simulink model "CTRL_UP_YAWACC_test"  (R2023b)
settings: Solver=VariableStepAuto  StartTime=0.0  StopTime=10.0  RelTol=1e-3
libraries: CTRL_UP_YAWACC x1
settings Model: Creator=blatak  LastModifiedBy=blatak

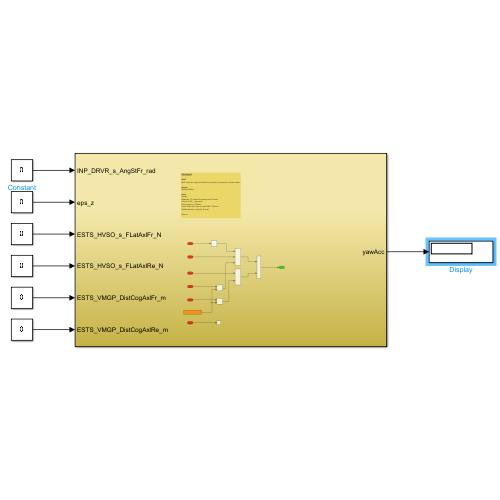
[thumbnail: Simulink's stored preview of the top-level diagram]
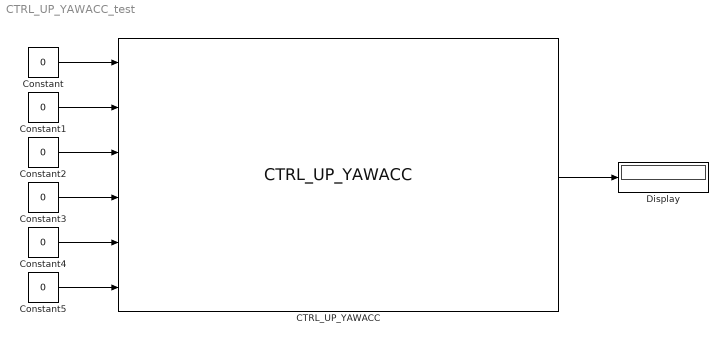
== system CTRL_UP_YAWACC_test ==
  CTRL_UP_YAWACC : CTRL_UP_YAWACC/CTRL_UP_YAWACC  SystemSampleTime=-1  VariantActivationTime=update diagram  AllowFlexibleInterface=on  Latency=0  AutoFrameSizeCalculation=off
  Constant{,1..5} (6 alike) : Constant  Value=0  OutDataTypeStr=single
  Display : Display
  wires:
  Constant/1 -> CTRL_UP_YAWACC/1
  Constant1/1 -> CTRL_UP_YAWACC/2
  Constant2/1 -> CTRL_UP_YAWACC/3
  Constant3/1 -> CTRL_UP_YAWACC/4
  Constant4/1 -> CTRL_UP_YAWACC/5
  Constant5/1 -> CTRL_UP_YAWACC/6
  CTRL_UP_YAWACC/1 -> Display/1
